simulink model "LKA_Lenkung_CarMaker_DSR_kombiniert_algSynth"  (Simulink 7.4)
settings: Solver=ode45  StartTime=0.0  StopTime=tend-1  FixedStep=0.01  RelTol=1e-3
libraries: library x4, simulink x3
settings Model: Creator=Georg  LastModifiedBy=Georg

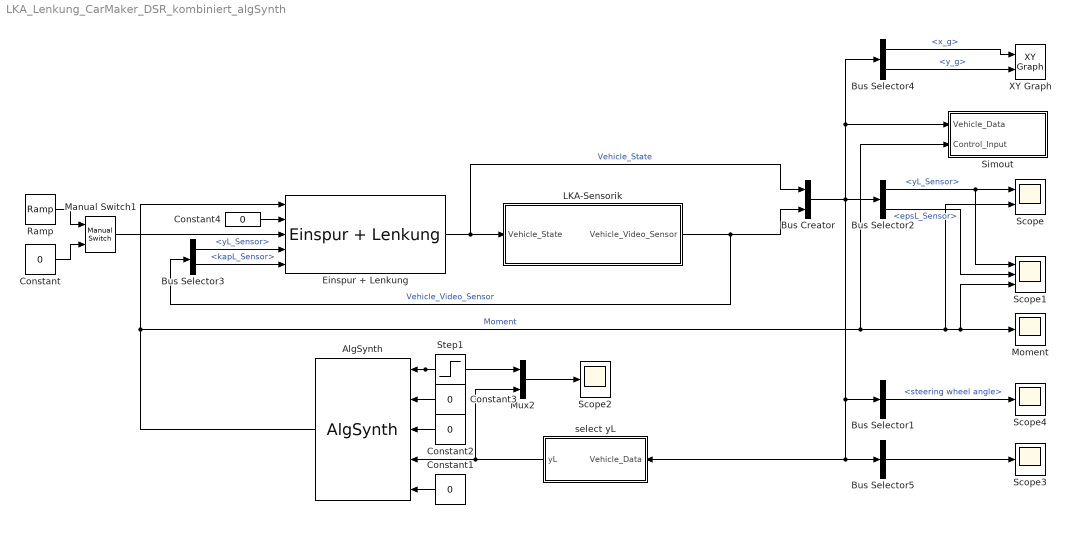
== system LKA_Lenkung_CarMaker_DSR_kombiniert_algSynth ==
  AlgSynth : library/LKA-Controller/AlgSynth  SystemSampleTime=-1
  Bus Creator : BusCreator  Inputs=2
  Bus Selector1 : BusSelector  OutputSignals=Vehicle_State.steering wheel angle
  Bus Selector2 : BusSelector  OutputSignals=Vehicle_Video_Sensor.yL_Sensor,Vehicle_Video_Sensor.epsL_Sensor
  Bus Selector3 : BusSelector  OutputSignals=yL_Sensor,kapL_Sensor
  Bus Selector4 : BusSelector  OutputSignals=Vehicle_State.x_g,Vehicle_State.y_g
  Bus Selector5 : BusSelector  OutputSignals=Vehicle_State.epsL_exactMdl,Vehicle_Video_Sensor.epsL_Sensor  OutputAsBus=on
  Constant{,1..4} (5 alike) : Constant  Value=0  OutDataType=fixdt(1, 16)  OutScaling=2^0
  Einspur + Lenkung : library/Vehicle Models/Einspur + Lenkung  SystemSampleTime=-1
  LKA-Sensorik : Subsystem  BlockChoice=Videosensorik
      settings: AttributesFormatString=%<BlockChoice>  TemplateBlock=library/LKA-Sensorik/LKA-Sensorik  MemberBlocks=Videosensorik
  Manual Switch1 : simulink/Signal Routing/Manual Switch  SystemSampleTime=-1  sw=0  action=0  varsize=off
  Moment : Scope
      settings: TimeRange=32.2  YMin=0.0002694  YMax=0.0002697  SaveName=ScopeData2
  Mux2 : Mux  Inputs=2
  Ramp : simulink/Sources/Ramp  SystemSampleTime=-1  slope=1  start=20  X0=0
  Scope : Scope  NumInputPorts=2
      settings: TimeRange=12.7664  YMin=-2.5e-006~-1e-005  YMax=3.25e-005~0.0002
  Scope1 : Scope  NumInputPorts=3
      settings: TimeRange=20  YMin=-5.5e-008~0.01711~-1.666e-008  YMax=5e-009~0.017145~-1.6565e-008
  Scope2 : Scope
      settings: TimeRange=5.66  YMin=0  YMax=1.05e-008  SaveName=ScopeData6
  Scope3 : Scope
      settings: YMin=0  YMax=0.035  SaveName=ScopeData3
  Scope4 : Scope
      settings: YMin=-0.005  YMax=0.09  SaveName=ScopeData4
  Simout : Subsystem
  Step1 : Step  Time=10  After=0  SampleTime=0
  XY Graph : simulink/Sinks/XY Graph  SystemSampleTime=-1  xmin=-100  xmax=700  ymin=-1  ymax=600  st=-1
  select yL : Subsystem  BlockChoice=yL_Sensor
      settings: AttributesFormatString=%<BlockChoice>  TemplateBlock=library/LKA-Sensorik/select yL  MemberBlocks=yL_Sensor,yL_exactMdl,yL_linMdl
  wires:
  Bus Selector4/1 -> XY Graph/1  "<x_g>"
  Bus Selector4/2 -> XY Graph/2  "<y_g>"
  Bus Selector2/1 -> Scope/1, Scope1/1  "<yL_Sensor>"
  Bus Selector2/2 -> Scope1/2  "<epsL_Sensor>"
  Einspur + Lenkung/1 -> LKA-Sensorik/1(Vehicle_State), Bus Creator/1  "Vehicle_State"
  LKA-Sensorik/1(Vehicle_Video_Sensor) -> Bus Creator/2, Bus Selector3/1  "Vehicle_Video_Sensor"
  Bus Creator/1 -> Bus Selector2/1, Bus Selector1/1, Bus Selector5/1, select yL/1(Vehicle_Data), Bus Selector4/1, Simout/1(Vehicle_Data)
  Bus Selector5/1 -> Scope3/1
  Bus Selector1/1 -> Scope4/1  "<steering wheel angle>"
  Constant/1 -> Manual Switch1/2
  Manual Switch1/1 -> Einspur + Lenkung/3
  Bus Selector3/1 -> Einspur + Lenkung/4  "<yL_Sensor>"
  Bus Selector3/2 -> Einspur + Lenkung/5  "<kapL_Sensor>"
  select yL/1(yL) -> Mux2/2, AlgSynth/4
  AlgSynth/1 -> Scope/2, Scope1/3, Moment/1, Simout/2(Control_Input), Einspur + Lenkung/1  "Moment"
  Mux2/1 -> Scope2/1
  Step1/1 -> Mux2/1, AlgSynth/1
  Constant3/1 -> AlgSynth/2
  Constant2/1 -> AlgSynth/3
  Constant1/1 -> AlgSynth/5
  Constant4/1 -> Einspur + Lenkung/2
  Ramp/1 -> Manual Switch1/1

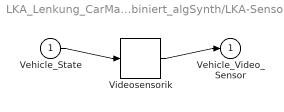
== system LKA_Lenkung_CarMaker_DSR_kombiniert_algSynth/LKA-Sensorik ==
  Vehicle_State : Inport
  Videosensorik : library/LKA-Sensorik/Videosensorik  SystemSampleTime=-1
  Vehicle_Video_Sensor : Outport
  wires:
  Vehicle_State/1 -> Videosensorik/1
  Videosensorik/1 -> Vehicle_Video_Sensor/1

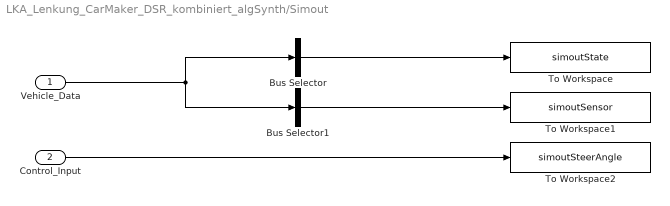
== system LKA_Lenkung_CarMaker_DSR_kombiniert_algSynth/Simout ==
  Vehicle_Data : Inport  OutDataType=fixdt(1, 16)  OutScaling=2^0
  Control_Input : Inport  Port=2  OutDataType=fixdt(1, 16)  OutScaling=2^0
  Bus Selector : BusSelector  OutputSignals=Vehicle_State  OutputAsBus=on
  Bus Selector1 : BusSelector  OutputSignals=Vehicle_Video_Sensor  OutputAsBus=on
  To Workspace : ToWorkspace  VariableName=simoutState  SampleTime=-1  SaveFormat=Structure With Time
  To Workspace1 : ToWorkspace  VariableName=simoutSensor  SampleTime=-1  SaveFormat=Structure With Time
  To Workspace2 : ToWorkspace  VariableName=simoutSteerAngle  SampleTime=-1  SaveFormat=Structure With Time
  wires:
  Vehicle_Data/1 -> Bus Selector1/1, Bus Selector/1
  Control_Input/1 -> To Workspace2/1
  Bus Selector/1 -> To Workspace/1
  Bus Selector1/1 -> To Workspace1/1

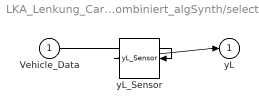
== system LKA_Lenkung_CarMaker_DSR_kombiniert_algSynth/select yL ==
  Vehicle_Data : Inport
  yL_Sensor : library/LKA-Sensorik/yL_Sensor  SystemSampleTime=-1
  yL : Outport
  wires:
  Vehicle_Data/1 -> yL_Sensor/1
  yL_Sensor/1 -> yL/1
